simulink model "at3_2"  (R2020a)
settings: Solver=VariableStepAuto  StartTime=0.0  StopTime=3.5  RelTol=1e-3
model workspace (MAT data in the model file):
  T = [1  0  0  0; 0  1  0  0; 0  0  1  0; 0  0  0  1]
  bd = 5
  kd = 10
  md = 1
  myFd = [0; 0; 5; 0; 0; 0]
  mybot = SerialLink
  mybot.name = 'mybot'
  mybot.gravity = [0; 0; 9.81]
  mybot.base = SE3
  mybot.base.data = [1  0  0  0; 0  1  0  0; 0  0  1  0; 0  0  0  1]
  mybot.tool = SE3
  mybot.tool.data = [1  0  0  0; 0  1  0  0; 0  0  1  0; 0  0  0  1]
  mybot.fast = 0
  mybot.delay = 0.1
  mybot.loop = 0
  mybot.n = 6
  mybot.links(1) = Link
  mybot.links(1).theta = 0
  mybot.links(1).d = 0.29333
  mybot.links(1).alpha = -1.57079632679
  mybot.links(1).a = 0.26667
  mybot.links(1).jointtype = 'R'
  mybot.links(1).mdh = 0
  mybot.links(1).offset = 0
  mybot.links(1).flip = 0
  mybot.links(1).m = 60.981037037
  mybot.links(1).r = [-0.139481333333 0.0867106666667 -0.0425993333333]
  mybot.links(1).I = [0.756881647671  0.0380732803951  -0.104663306798; 0.0380732803951  1.31862233218  -0.0252104658436; -0.104663306798  -0.0252104658436  1.48229918249]
  mybot.links(1).Jm = 0
  mybot.links(1).B = 0
  mybot.links(1).Tc = [0 0]
  mybot.links(1).G = 0
  mybot.links(1).qlim = [-3.14159265359 3.14159265359]
  mybot.links(2) = Link
  mybot.links(2).theta = 0
  mybot.links(2).d = 0
  mybot.links(2).alpha = 0
  mybot.links(2).a = 0.666666666667
  mybot.links(2).jointtype = 'R'
  mybot.links(2).mdh = 0
  mybot.links(2).offset = -1.57079632679
  mybot.links(2).flip = 0
  mybot.links(2).m = 30.4687407407
  mybot.links(2).r = [-0.364482 0.031008 -0.203550666667]
  mybot.links(2).I = [0.445067283621  -0.108967727539  0.582977155556; -0.108967727539  5.764327397  -0.00631798241975; 0.582977155556  -0.00631798241975  5.74215637531]
  mybot.links(2).Jm = 0
  mybot.links(2).B = 0
  mybot.links(2).Tc = [0 0]
  mybot.links(2).G = 0
  mybot.links(2).qlim = [-1.24756134933 1.28316606607]
  mybot.links(3) = Link
  mybot.links(3).theta = 0
  mybot.links(3).d = 0
  mybot.links(3).alpha = -1.57079632679
  mybot.links(3).a = 0
  mybot.links(3).jointtype = 'R'
  mybot.links(3).mdh = 0
  mybot.links(3).offset = 0
  mybot.links(3).flip = 0
  mybot.links(3).m = 79.3111111111
  mybot.links(3).r = [-0.00110933333333 0.0488613333333 0.203686]
  mybot.links(3).I = [1.64625289455  -0.0104833337942  0.0982028045432; -0.0104833337942  1.62048570864  -0.0496952560988; 0.0982028045432  -0.0496952560988  0.173149863111]
  mybot.links(3).Jm = 0
  mybot.links(3).B = 0
  mybot.links(3).Tc = [0 0]
  mybot.links(3).G = 0
  mybot.links(3).qlim = [-3.56431139842 1.14807758196]
  mybot.links(4) = Link
  mybot.links(4).theta = 0
  mybot.links(4).d = 0.87133
  mybot.links(4).alpha = 1.57079632679
  mybot.links(4).a = 0
  mybot.links(4).jointtype = 'R'
  mybot.links(4).mdh = 0
  mybot.links(4).offset = 0
  mybot.links(4).flip = 0
  mybot.links(4).m = 7.42785185185
  mybot.links(4).r = [0 -0.114642 -0.0563753333333]
  mybot.links(4).I = [0.0760047099259  -0.00573300266667  8.43277695473e-05; -0.00573300266667  0.0244535510123  -0.000540736395062; 8.43277695473e-05  -0.000540736395062  0.0768069846914]
  mybot.links(4).Jm = 0
  mybot.links(4).B = 0
  mybot.links(4).Tc = [0 0]
  mybot.links(4).G = 0
  mybot.links(4).qlim = [-3.14159265359 3.14159265359]
  mybot.links(5) = Link
  mybot.links(5).theta = 0
  mybot.links(5).d = 0
  mybot.links(5).alpha = -1.57079632679
  mybot.links(5).a = 0
  mybot.links(5).jointtype = 'R'
  mybot.links(5).mdh = 0
  mybot.links(5).offset = 0
  mybot.links(5).flip = 0
  mybot.links(5).m = 3.22814814815
  mybot.links(5).r = [0 0.055874 0.009464]
  mybot.links(5).I = [0.0620193424856  -0.00336486123457  0.00258873902881; -0.00336486123457  0.0425072813827  -0.00932130199177; 0.00258873902881  -0.00932130199177  0.042955055144]
  mybot.links(5).Jm = 0
  mybot.links(5).B = 0
  mybot.links(5).Tc = [0 0]
  mybot.links(5).G = 0
  mybot.links(5).qlim = [-1.91986217719 1.91986217719]
  mybot.links(6) = Link
  mybot.links(6).theta = 0
  mybot.links(6).d = 0.40667
  mybot.links(6).alpha = 0
  mybot.links(6).a = 0
  mybot.links(6).jointtype = 'R'
  mybot.links(6).mdh = 0
  mybot.links(6).offset = 0
  mybot.links(6).flip = 0
  mybot.links(6).m = 0.993777777778
  mybot.links(6).r = [7.33333333333e-06 0.0546666666667 -0.0859013333333]
  mybot.links(6).I = [0.00060011417284  0  0; 0  0.000924736395062  0; 0  0  0.000554118716049]
  mybot.links(6).Jm = 0
  mybot.links(6).B = 0
  mybot.links(6).Tc = [0 0]
  mybot.links(6).G = 0
  mybot.links(6).qlim = [-3.14159265359 3.14159265359]
  mybot.mdh = 0
values from neighbouring files (symbols this model uses):
  Fd2 = [0 0 5 0 0 0]'    [main.m]
  Fd3 = [0 0 0 0 0 0]'    [main.m]
  m = [171.459 140.993 94.498 31.976 31.091 0.606]    [I.mat]    (also in main.m = [205.811,102.832,267.675,25.069,10.895,3.354]; maincircle.m = [205.811,102.832,267.675,25.069,10.895,3.354])
undefined symbols (not defined in the file or in its folder): X, Y, Z
libraries: sm_lib x76, nesl_utility x31, simulink_extras x21, roblocks x16, simulink x7
(part 1 of 3)
settings Model: PauseTimes=1.625  Creator=93548  LastModifiedBy=93548

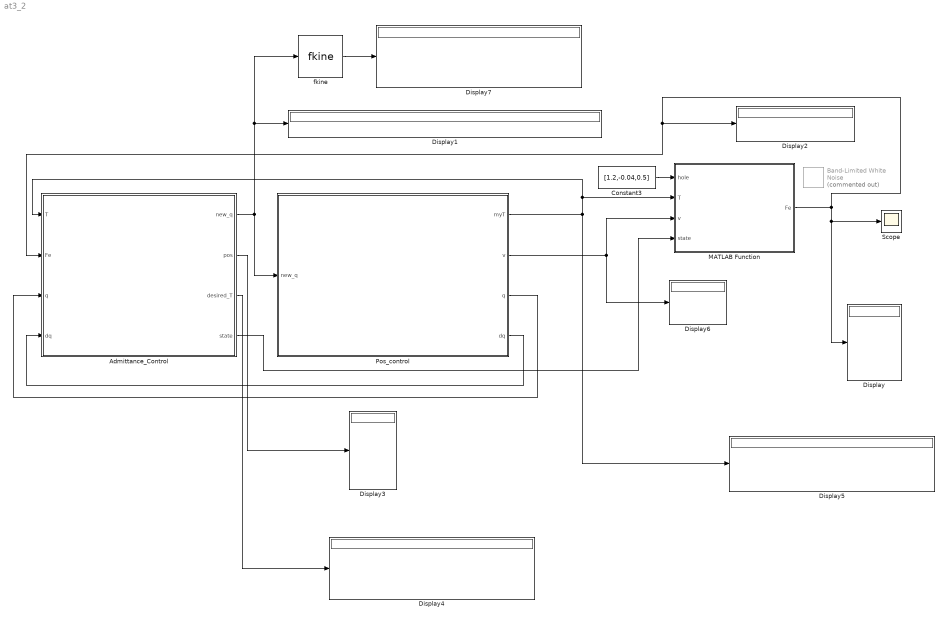
== system at3_2 ==
  Admittance_Control : Subsystem
  Band-Limited White Noise : simulink/Sources/Band-Limited White Noise  Commented=on  Cov=0.00001*ones(1,6)  Ts=0.01  seed=[23341 2221 2342 4533 53 123]
  Constant3 : Constant  Value=[1.2,-0.04,0.5]
  Display{,1..7} (8 alike) : Display
  MATLAB Function : MATLAB Function  TreatAsAtomicUnit=on
  Pos_control : Subsystem
  Scope : Scope
  fkine : roblocks/Arm/fkine  robot=mybot
  wires:
  Admittance_Control/3(desired_T) -> Display4/1
  Pos_control/3(q) -> Admittance_Control/3(q)
  MATLAB Function/1(Fe) -> Display2/1, Admittance_Control/2(Fe), Scope/1, Display/1
  Pos_control/1(myT) -> MATLAB Function/2(T), Admittance_Control/1(T), Display5/1
  Pos_control/4(dq) -> Admittance_Control/4(dq)
  Constant3/1 -> MATLAB Function/1(hole)
  Admittance_Control/1(new_q) -> Pos_control/1(new_q), fkine/1, Display1/1
  Admittance_Control/2(pos) -> Display3/1
  Pos_control/2(v) -> MATLAB Function/3(v), Display6/1
  fkine/1 -> Display7/1
  Admittance_Control/4(state) -> MATLAB Function/4(state)

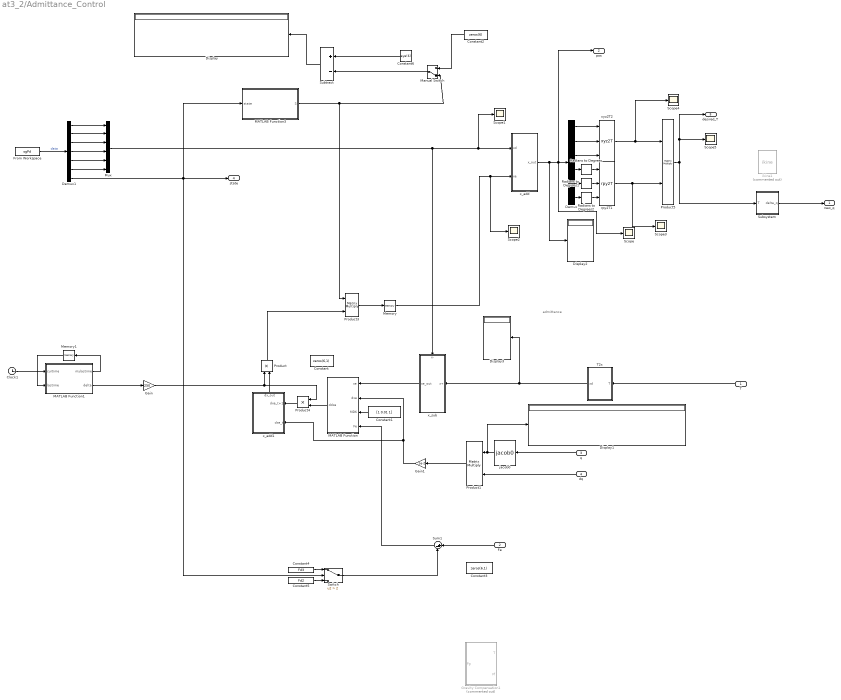
== system at3_2/Admittance_Control ==
  note: admittance
  T : Inport  InitFcn=T=eye(4)
  Fe : Inport  Port=2
  q : Inport  Port=3
  dq : Inport  Port=4
  Clock1 : Clock
  Constant : Constant  Value=zeros(6,1)
  Constant1 : Constant  Value=[1 0.01 1]
  Constant2 : Constant  Value=zeros(6)
  Constant3 : Constant  Value=zeros(6,1)
  Constant4 : Constant  Value=Fd3
  Constant5 : Constant  Value=Fd2
  Constant6 : Constant  Value=eye(6)
  Demux : Demux  Outputs=6
  Demux1 : Demux  Outputs=7
  Display{,1..3} (4 alike) : Display
  From Workspace : FromWorkspace  VariableName=sgPd
  Gain : Gain  Gain=250
  Gain1 : Gain  Gain=1e-2
  Gravity Compensation1 : MATLAB Function  Commented=on  TreatAsAtomicUnit=on
  MATLAB Function : MATLAB Function  TreatAsAtomicUnit=on
  MATLAB Function1 : MATLAB Function  TreatAsAtomicUnit=on
  MATLAB Function3 : MATLAB Function  TreatAsAtomicUnit=on
  Manual Switch : ManualSwitch  CurrentSetting=0
  Memory : Memory  InitialCondition=zeros(6,1)
  Memory1 : Memory
  Mux : Mux  Inputs=6
  Product : Product
  Product1 : Product  Multiplication=Matrix(*)
  Product3 : Product  Multiplication=Matrix(*)
  Product4 : Product
  Product5 : Product  Multiplication=Matrix(*)
  Radians to Degrees : simulink_extras/Transformations/Radians to Degrees
  Radians to Degrees1 : simulink_extras/Transformations/Radians to Degrees
  Radians to Degrees2 : simulink_extras/Transformations/Radians to Degrees
  Scope{,1..5} (6 alike) : Scope
  Subsystem : Subsystem
  Subtract : Sum  Inputs=+-
  Sum1 : Sum  Inputs=|+-
  Switch : Switch  Criteria=u2 > Threshold  Threshold=2
  T2x : Subsystem
  ikine1 : roblocks/Arm/ikine  Commented=on  robot=mybot  q0=zeros(6,1)  M=[1 1 1 1 1 1]  pinv=off  options={}
  "jacob0 " : roblocks/Arm/jacob0   robot=mybot
  rpy2T1 : roblocks/Toolbox/rpy2T  sequence=XYZ  degrees=off
  x_add : Subsystem
  x_add1 : Subsystem
      settings: PortSchema="{\"entries\":[{\"content\":{\"sides\":[{\"content\":{\"connectorIds\":[\"In1\",\"In2\"]},\"type\":\"ConnectorPlacement.EquallySpacedRectSide\",\"uuid\":\"360d4010-1b97-427a-9903-25c88b23e70b\"},{\"content\":{\"connectorIds\":[],\"side\":\"RIGHT\"},\"type\":\"ConnectorPlacement.EquallySpacedRectSide\",\"uuid\":\"9a31a209-5194-4c7d-8d7e-c14204494445\"},{\"content\":{\"connectorIds\":[\"Out1\"],\"side\":\"TOP\"},\"type\":\"ConnectorPlacement.EquallySpacedRectSide\",\"uuid\":\"bbbce9f7-61ee-4f1f-a5ce-85863fd91b3c\"}]},\"type\":\"ConnectorPlacement.EquallySpacedConnector\",\"uuid\":\"e93273eb-05a0-482b-8f1c-7b726ecfc3e6\"}],\"packageUris\":[\"http://schema.mathworks.com/mf0/Connector/19700101\"],\"version\":\"1.0\"}"
  x_sub : Subsystem
      settings: PortSchema="{\"entries\":[{\"content\":{\"sides\":[{\"content\":{\"connectorIds\":[\"In1\"]},\"type\":\"ConnectorPlacement.EquallySpacedRectSide\",\"uuid\":\"dec81ac2-0bd0-410d-a885-3af3e0ce6e73\"},{\"content\":{\"connectorIds\":[\"Out1\"],\"side\":\"RIGHT\"},\"type\":\"ConnectorPlacement.EquallySpacedRectSide\",\"uuid\":\"6534a841-e66b-4c1b-a3eb-8f152edb689c\"},{\"content\":{\"connectorIds\":[\"In2\"],\"side\":\"TOP\"},\"type\":\"ConnectorPlacement.EquallySpacedRectSide\",\"uuid\":\"16d8580e-7ffb-477c-bb08-41121949b294\"}]},\"type\":\"ConnectorPlacement.EquallySpacedConnector\",\"uuid\":\"cf84df31-fda1-43e7-8245-e4491d5279cc\"}],\"packageUris\":[\"http://schema.mathworks.com/mf0/Connector/19700101\"],\"version\":\"1.0\"}"
  xyz2T2 : roblocks/Toolbox/xyz2T
  new_q : Outport
  pos : Outport  Port=2
  desired_T : Outport  Port=3
  state : Outport  Port=4
  wires:
  Fe/1 -> Sum1/1
  rpy2T1/1 -> Product5/2, Scope3/1
  Demux/1 -> xyz2T2/1
  Demux/2 -> xyz2T2/2
  Demux/3 -> xyz2T2/3
  Demux/4 -> Radians to Degrees/1
  Demux/5 -> Radians to Degrees1/1
  Demux/6 -> Radians to Degrees2/1
  Constant6/1 -> Subtract/1
  T2x/1(xd) -> Display3/1, x_sub/1(x+)
  "jacob0 "/1 -> Display1/1, Product1/1
  x_sub/1(xe_out) -> MATLAB Function/1(xe)
  Constant1/1 -> MATLAB Function/3(MDK)
  MATLAB Function/1(ddxe) -> Product4/2
  x_add1/1(dx_out) -> Product/2
  Subtract/1 -> Display/1
  Mux/1 -> x_sub/2(x-), Scope1/1, x_add/1(xd)
  Manual Switch/1 -> Subtract/2
  MATLAB Function3/1(S) -> Manual Switch/2, Product3/1
  Constant2/1 -> Manual Switch/1
  T/1 -> T2x/1(T)
  Radians to Degrees/1 -> rpy2T1/1
  Radians to Degrees1/1 -> rpy2T1/2
  Radians to Degrees2/1 -> rpy2T1/3
  From Workspace/1 -> Demux1/1  "data"
  Demux1/6 -> Mux/6
  Demux1/5 -> Mux/5
  Demux1/3 -> Mux/3
  Demux1/4 -> Mux/4
  Demux1/2 -> Mux/2
  Demux1/1 -> Mux/1
  Demux1/7 -> MATLAB Function3/1(state), state/1, Switch/2
  x_add/1(x_out) -> Scope/1, Demux/1, pos/1, Display2/1
  Product5/1 -> Scope5/1, desired_T/1, Subsystem/1(T)
  Product/1 -> Product3/2
  q/1 -> "jacob0 "/1
  dq/1 -> Product1/2
  Product3/1 -> Memory/1
  Memory/1 -> Scope2/1, x_add/2(xe)
  Sum1/1 -> MATLAB Function/4(Fe)
  Constant4/1 -> Switch/1
  Constant5/1 -> Switch/3
  Switch/1 -> Sum1/2
  MATLAB Function1/2(delta) -> Gain/1
  MATLAB Function1/1(mylastime) -> Memory1/1
  Clock1/1 -> MATLAB Function1/1(curtime)
  Memory1/1 -> MATLAB Function1/2(lastime)
  Product4/1 -> x_add1/1(dxe_t+1)
  Subsystem/1(delta_q) -> new_q/1
  xyz2T2/1 -> Scope4/1, Product5/1
  Gain/1 -> Product4/1, Product/1
  Gain1/1 -> MATLAB Function/2(dxe), x_add1/2(dxe_t)
  Product1/1 -> Gain1/1

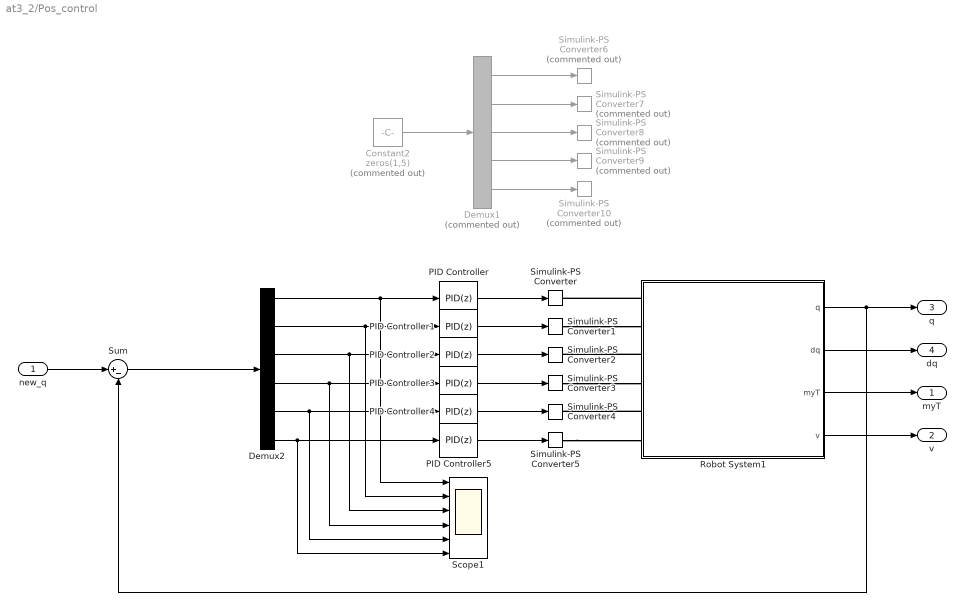
== system at3_2/Pos_control ==
  new_q : Inport
  Constant2 : Constant  Commented=on  Value=zeros(1,5)
  Demux1 : Demux  Commented=on  Outputs=5
  Demux2 : Demux  Outputs=6
  PID Controller : simulink/Continuous/PID Controller  Controller=PID  Form=Parallel  TimeDomain=Discrete-time  UseExternalTs=off  SampleTime=-1  IntegratorMethod=Forward Euler  FilterMethod=Forward Euler  ControllerParametersSource=internal  P=4465.98498018288  I=7608.36685462562  D=641.613681305102  UseFilter=on  N=345.506450530319  TunerSelectOption=Transfer Function Based (PID Tuner App)  InitialConditionSource=internal  InitialConditionForIntegrator=0  InitialConditionForFilter=0  DifferentiatorICPrevScaledInput=0  ExternalReset=none  TrackingMode=off  Kt=1  LimitOutput=off  UpperSaturationLimit=inf  LowerSaturationLimit=-inf  LinearizeAsGain=on  AntiWindupMode=none  Kb=1  POutMin=[]  POutMax=[]  IOutMin=[]  IOutMax=[]  DOutMin=[]  DOutMax=[]  NOutMin=[]  NOutMax=[]  SumOutMin=[]  SumOutMax=[]  SaturationOutMin=[]  SaturationOutMax=[]  PParamMin=[]  PParamMax=[]  IParamMin=[]  IParamMax=[]  DParamMin=[]  DParamMax=[]  NParamMin=[]  NParamMax=[]  KbParamMin=[]  KbParamMax=[]  KtParamMin=[]  KtParamMax=[]  KbOutMin=[]  KbOutMax=[]  KtOutMin=[]  KtOutMax=[]  IntegratorOutMin=[]  IntegratorOutMax=[]  FilterOutMin=[]  FilterOutMax=[]  SumI1OutMin=[]  SumI1OutMax=[]  SumI2OutMin=[]  SumI2OutMax=[]  SumI3OutMin=[]  SumI3OutMax=[]  SumI4OutMin=[]  SumI4OutMax=[]  SumDOutMin=[]  SumDOutMax=[]  DifferentiatorOutMin=[]  DifferentiatorOutMax=[]  FilterDiffOutCoefMin=[]  FilterDiffOutCoefMax=[]  ReciprocalOutMin=[]  ReciprocalOutMax=[]  SumDenOutMin=[]  SumDenOutMax=[]  SumNumOutMin=[]  SumNumOutMax=[]  DivideOutMin=[]  DivideOutMax=[]  UdiffTsProdOutMin=[]  UdiffTsProdOutMax=[]  NTsProdOutMin=[]  NTsProdOutMax=[]  UintegralTsProdOutMin=[]  UintegralTsProdOutMax=[]  UngainTsProdOutMin=[]  UngainTsProdOutMax=[]  IntegratorContinuousStateAttributes=''  IntegratorStateMustResolveToSignalObject=off  IntegratorRTWStateStorageClass=Auto  FilterContinuousStateAttributes=''  FilterStateMustResolveToSignalObject=off  FilterRTWStateStorageClass=Auto  ParallelPVariant=InternalParameters  IdealPVariant=Disabled  IVariant=InternalParameters  DVariant=InternalParameters  IntegratorVariant=Discrete  SatVariant=Disabled  AWVariant=Passthrough  PCopyVariant=Disabled  TRVariant=Disabled  FdbkBlocksVariant=Forward  IdealPFdbkVariant=Disabled  SatFdbkVariant=Disabled  DerivativeFilterVariant=ForwardEulerFilter  NVariant=InternalParameters  NCopyVariant=Disabled  FilterICVariant=InternalICsFilter  IntegratorICVariant=InternalICs  ExternalResetVariant=Disabled  TRSumVariant=Passthrough  SumFdbkVariant=Disabled  SumVariant=Sum_PID  TsampFilterVariant=InternalTs  TsampNgainVariant=Passthrough  TsampIntegralVariant=Passthrough
  PID Controller1 : simulink/Continuous/PID Controller  Controller=PID  Form=Parallel  TimeDomain=Discrete-time  UseExternalTs=off  SampleTime=-1  IntegratorMethod=Forward Euler  FilterMethod=Forward Euler  ControllerParametersSource=internal  P=16138.220391969  I=29003.8058546243  D=1312.1656601102  UseFilter=on  N=1517.01833251505  TunerSelectOption=Transfer Function Based (PID Tuner App)  InitialConditionSource=internal  InitialConditionForIntegrator=0  InitialConditionForFilter=0  DifferentiatorICPrevScaledInput=0  ExternalReset=none  TrackingMode=off  Kt=1  LimitOutput=off  UpperSaturationLimit=inf  LowerSaturationLimit=-inf  LinearizeAsGain=on  AntiWindupMode=none  Kb=1  POutMin=[]  POutMax=[]  IOutMin=[]  IOutMax=[]  DOutMin=[]  DOutMax=[]  NOutMin=[]  NOutMax=[]  SumOutMin=[]  SumOutMax=[]  SaturationOutMin=[]  SaturationOutMax=[]  PParamMin=[]  PParamMax=[]  IParamMin=[]  IParamMax=[]  DParamMin=[]  DParamMax=[]  NParamMin=[]  NParamMax=[]  KbParamMin=[]  KbParamMax=[]  KtParamMin=[]  KtParamMax=[]  KbOutMin=[]  KbOutMax=[]  KtOutMin=[]  KtOutMax=[]  IntegratorOutMin=[]  IntegratorOutMax=[]  FilterOutMin=[]  FilterOutMax=[]  SumI1OutMin=[]  SumI1OutMax=[]  SumI2OutMin=[]  SumI2OutMax=[]  SumI3OutMin=[]  SumI3OutMax=[]  SumI4OutMin=[]  SumI4OutMax=[]  SumDOutMin=[]  SumDOutMax=[]  DifferentiatorOutMin=[]  DifferentiatorOutMax=[]  FilterDiffOutCoefMin=[]  FilterDiffOutCoefMax=[]  ReciprocalOutMin=[]  ReciprocalOutMax=[]  SumDenOutMin=[]  SumDenOutMax=[]  SumNumOutMin=[]  SumNumOutMax=[]  DivideOutMin=[]  DivideOutMax=[]  UdiffTsProdOutMin=[]  UdiffTsProdOutMax=[]  NTsProdOutMin=[]  NTsProdOutMax=[]  UintegralTsProdOutMin=[]  UintegralTsProdOutMax=[]  UngainTsProdOutMin=[]  UngainTsProdOutMax=[]  IntegratorContinuousStateAttributes=''  IntegratorStateMustResolveToSignalObject=off  IntegratorRTWStateStorageClass=Auto  FilterContinuousStateAttributes=''  FilterStateMustResolveToSignalObject=off  FilterRTWStateStorageClass=Auto  ParallelPVariant=InternalParameters  IdealPVariant=Disabled  IVariant=InternalParameters  DVariant=InternalParameters  IntegratorVariant=Discrete  SatVariant=Disabled  AWVariant=Passthrough  PCopyVariant=Disabled  TRVariant=Disabled  FdbkBlocksVariant=Forward  IdealPFdbkVariant=Disabled  SatFdbkVariant=Disabled  DerivativeFilterVariant=ForwardEulerFilter  NVariant=InternalParameters  NCopyVariant=Disabled  FilterICVariant=InternalICsFilter  IntegratorICVariant=InternalICs  ExternalResetVariant=Disabled  TRSumVariant=Passthrough  SumFdbkVariant=Disabled  SumVariant=Sum_PID  TsampFilterVariant=InternalTs  TsampNgainVariant=Passthrough  TsampIntegralVariant=Passthrough
  PID Controller2 : simulink/Continuous/PID Controller  Controller=PID  Form=Parallel  TimeDomain=Discrete-time  UseExternalTs=off  SampleTime=-1  IntegratorMethod=Forward Euler  FilterMethod=Forward Euler  ControllerParametersSource=internal  P=1649.40066842326  I=2863.75247346737  D=182.018728238073  UseFilter=on  N=172.788597852014  TunerSelectOption=Transfer Function Based (PID Tuner App)  InitialConditionSource=internal  InitialConditionForIntegrator=0  InitialConditionForFilter=0  DifferentiatorICPrevScaledInput=0  ExternalReset=none  TrackingMode=off  Kt=1  LimitOutput=off  UpperSaturationLimit=inf  LowerSaturationLimit=-inf  LinearizeAsGain=on  AntiWindupMode=none  Kb=1  POutMin=[]  POutMax=[]  IOutMin=[]  IOutMax=[]  DOutMin=[]  DOutMax=[]  NOutMin=[]  NOutMax=[]  SumOutMin=[]  SumOutMax=[]  SaturationOutMin=[]  SaturationOutMax=[]  PParamMin=[]  PParamMax=[]  IParamMin=[]  IParamMax=[]  DParamMin=[]  DParamMax=[]  NParamMin=[]  NParamMax=[]  KbParamMin=[]  KbParamMax=[]  KtParamMin=[]  KtParamMax=[]  KbOutMin=[]  KbOutMax=[]  KtOutMin=[]  KtOutMax=[]  IntegratorOutMin=[]  IntegratorOutMax=[]  FilterOutMin=[]  FilterOutMax=[]  SumI1OutMin=[]  SumI1OutMax=[]  SumI2OutMin=[]  SumI2OutMax=[]  SumI3OutMin=[]  SumI3OutMax=[]  SumI4OutMin=[]  SumI4OutMax=[]  SumDOutMin=[]  SumDOutMax=[]  DifferentiatorOutMin=[]  DifferentiatorOutMax=[]  FilterDiffOutCoefMin=[]  FilterDiffOutCoefMax=[]  ReciprocalOutMin=[]  ReciprocalOutMax=[]  SumDenOutMin=[]  SumDenOutMax=[]  SumNumOutMin=[]  SumNumOutMax=[]  DivideOutMin=[]  DivideOutMax=[]  UdiffTsProdOutMin=[]  UdiffTsProdOutMax=[]  NTsProdOutMin=[]  NTsProdOutMax=[]  UintegralTsProdOutMin=[]  UintegralTsProdOutMax=[]  UngainTsProdOutMin=[]  UngainTsProdOutMax=[]  IntegratorContinuousStateAttributes=''  IntegratorStateMustResolveToSignalObject=off  IntegratorRTWStateStorageClass=Auto  FilterContinuousStateAttributes=''  FilterStateMustResolveToSignalObject=off  FilterRTWStateStorageClass=Auto  ParallelPVariant=InternalParameters  IdealPVariant=Disabled  IVariant=InternalParameters  DVariant=InternalParameters  IntegratorVariant=Discrete  SatVariant=Disabled  AWVariant=Passthrough  PCopyVariant=Disabled  TRVariant=Disabled  FdbkBlocksVariant=Forward  IdealPFdbkVariant=Disabled  SatFdbkVariant=Disabled  DerivativeFilterVariant=ForwardEulerFilter  NVariant=InternalParameters  NCopyVariant=Disabled  FilterICVariant=InternalICsFilter  IntegratorICVariant=InternalICs  ExternalResetVariant=Disabled  TRSumVariant=Passthrough  SumFdbkVariant=Disabled  SumVariant=Sum_PID  TsampFilterVariant=InternalTs  TsampNgainVariant=Passthrough  TsampIntegralVariant=Passthrough
  PID Controller3 : simulink/Continuous/PID Controller  Controller=PID  Form=Parallel  TimeDomain=Discrete-time  UseExternalTs=off  SampleTime=-1  IntegratorMethod=Forward Euler  FilterMethod=Forward Euler  ControllerParametersSource=internal  P=14.6989445468851  I=23.6851292927488  D=1.1771070717056  UseFilter=on  N=1533.69648335729  TunerSelectOption=Transfer Function Based (PID Tuner App)  InitialConditionSource=internal  InitialConditionForIntegrator=0  InitialConditionForFilter=0  DifferentiatorICPrevScaledInput=0  ExternalReset=none  TrackingMode=off  Kt=1  LimitOutput=off  UpperSaturationLimit=inf  LowerSaturationLimit=-inf  LinearizeAsGain=on  AntiWindupMode=none  Kb=1  POutMin=[]  POutMax=[]  IOutMin=[]  IOutMax=[]  DOutMin=[]  DOutMax=[]  NOutMin=[]  NOutMax=[]  SumOutMin=[]  SumOutMax=[]  SaturationOutMin=[]  SaturationOutMax=[]  PParamMin=[]  PParamMax=[]  IParamMin=[]  IParamMax=[]  DParamMin=[]  DParamMax=[]  NParamMin=[]  NParamMax=[]  KbParamMin=[]  KbParamMax=[]  KtParamMin=[]  KtParamMax=[]  KbOutMin=[]  KbOutMax=[]  KtOutMin=[]  KtOutMax=[]  IntegratorOutMin=[]  IntegratorOutMax=[]  FilterOutMin=[]  FilterOutMax=[]  SumI1OutMin=[]  SumI1OutMax=[]  SumI2OutMin=[]  SumI2OutMax=[]  SumI3OutMin=[]  SumI3OutMax=[]  SumI4OutMin=[]  SumI4OutMax=[]  SumDOutMin=[]  SumDOutMax=[]  DifferentiatorOutMin=[]  DifferentiatorOutMax=[]  FilterDiffOutCoefMin=[]  FilterDiffOutCoefMax=[]  ReciprocalOutMin=[]  ReciprocalOutMax=[]  SumDenOutMin=[]  SumDenOutMax=[]  SumNumOutMin=[]  SumNumOutMax=[]  DivideOutMin=[]  DivideOutMax=[]  UdiffTsProdOutMin=[]  UdiffTsProdOutMax=[]  NTsProdOutMin=[]  NTsProdOutMax=[]  UintegralTsProdOutMin=[]  UintegralTsProdOutMax=[]  UngainTsProdOutMin=[]  UngainTsProdOutMax=[]  IntegratorContinuousStateAttributes=''  IntegratorStateMustResolveToSignalObject=off  IntegratorRTWStateStorageClass=Auto  FilterContinuousStateAttributes=''  FilterStateMustResolveToSignalObject=off  FilterRTWStateStorageClass=Auto  ParallelPVariant=InternalParameters  IdealPVariant=Disabled  IVariant=InternalParameters  DVariant=InternalParameters  IntegratorVariant=Discrete  SatVariant=Disabled  AWVariant=Passthrough  PCopyVariant=Disabled  TRVariant=Disabled  FdbkBlocksVariant=Forward  IdealPFdbkVariant=Disabled  SatFdbkVariant=Disabled  DerivativeFilterVariant=ForwardEulerFilter  NVariant=InternalParameters  NCopyVariant=Disabled  FilterICVariant=InternalICsFilter  IntegratorICVariant=InternalICs  ExternalResetVariant=Disabled  TRSumVariant=Passthrough  SumFdbkVariant=Disabled  SumVariant=Sum_PID  TsampFilterVariant=InternalTs  TsampNgainVariant=Passthrough  TsampIntegralVariant=Passthrough
  PID Controller4 : simulink/Continuous/PID Controller  Controller=PID  Form=Parallel  TimeDomain=Discrete-time  UseExternalTs=off  SampleTime=-1  IntegratorMethod=Forward Euler  FilterMethod=Forward Euler  ControllerParametersSource=internal  P=98.6724069978625  I=118.426367034708  D=4.05904729962159  UseFilter=on  N=1784.33996524078  TunerSelectOption=Transfer Function Based (PID Tuner App)  InitialConditionSource=internal  InitialConditionForIntegrator=0  InitialConditionForFilter=0  DifferentiatorICPrevScaledInput=0  ExternalReset=none  TrackingMode=off  Kt=1  LimitOutput=off  UpperSaturationLimit=inf  LowerSaturationLimit=-inf  LinearizeAsGain=on  AntiWindupMode=none  Kb=1  POutMin=[]  POutMax=[]  IOutMin=[]  IOutMax=[]  DOutMin=[]  DOutMax=[]  NOutMin=[]  NOutMax=[]  SumOutMin=[]  SumOutMax=[]  SaturationOutMin=[]  SaturationOutMax=[]  PParamMin=[]  PParamMax=[]  IParamMin=[]  IParamMax=[]  DParamMin=[]  DParamMax=[]  NParamMin=[]  NParamMax=[]  KbParamMin=[]  KbParamMax=[]  KtParamMin=[]  KtParamMax=[]  KbOutMin=[]  KbOutMax=[]  KtOutMin=[]  KtOutMax=[]  IntegratorOutMin=[]  IntegratorOutMax=[]  FilterOutMin=[]  FilterOutMax=[]  SumI1OutMin=[]  SumI1OutMax=[]  SumI2OutMin=[]  SumI2OutMax=[]  SumI3OutMin=[]  SumI3OutMax=[]  SumI4OutMin=[]  SumI4OutMax=[]  SumDOutMin=[]  SumDOutMax=[]  DifferentiatorOutMin=[]  DifferentiatorOutMax=[]  FilterDiffOutCoefMin=[]  FilterDiffOutCoefMax=[]  ReciprocalOutMin=[]  ReciprocalOutMax=[]  SumDenOutMin=[]  SumDenOutMax=[]  SumNumOutMin=[]  SumNumOutMax=[]  DivideOutMin=[]  DivideOutMax=[]  UdiffTsProdOutMin=[]  UdiffTsProdOutMax=[]  NTsProdOutMin=[]  NTsProdOutMax=[]  UintegralTsProdOutMin=[]  UintegralTsProdOutMax=[]  UngainTsProdOutMin=[]  UngainTsProdOutMax=[]  IntegratorContinuousStateAttributes=''  IntegratorStateMustResolveToSignalObject=off  IntegratorRTWStateStorageClass=Auto  FilterContinuousStateAttributes=''  FilterStateMustResolveToSignalObject=off  FilterRTWStateStorageClass=Auto  ParallelPVariant=InternalParameters  IdealPVariant=Disabled  IVariant=InternalParameters  DVariant=InternalParameters  IntegratorVariant=Discrete  SatVariant=Disabled  AWVariant=Passthrough  PCopyVariant=Disabled  TRVariant=Disabled  FdbkBlocksVariant=Forward  IdealPFdbkVariant=Disabled  SatFdbkVariant=Disabled  DerivativeFilterVariant=ForwardEulerFilter  NVariant=InternalParameters  NCopyVariant=Disabled  FilterICVariant=InternalICsFilter  IntegratorICVariant=InternalICs  ExternalResetVariant=Disabled  TRSumVariant=Passthrough  SumFdbkVariant=Disabled  SumVariant=Sum_PID  TsampFilterVariant=InternalTs  TsampNgainVariant=Passthrough  TsampIntegralVariant=Passthrough
  PID Controller5 : simulink/Continuous/PID Controller  Controller=PID  Form=Parallel  TimeDomain=Discrete-time  UseExternalTs=off  SampleTime=-1  IntegratorMethod=Forward Euler  FilterMethod=Forward Euler  ControllerParametersSource=internal  P=1.57423793511941  I=4.99903335998905  D=0.109727091124155  UseFilter=on  N=1702.33251187192  TunerSelectOption=Transfer Function Based (PID Tuner App)  InitialConditionSource=internal  InitialConditionForIntegrator=0  InitialConditionForFilter=0  DifferentiatorICPrevScaledInput=0  ExternalReset=none  TrackingMode=off  Kt=1  LimitOutput=off  UpperSaturationLimit=inf  LowerSaturationLimit=-inf  LinearizeAsGain=on  AntiWindupMode=none  Kb=1  POutMin=[]  POutMax=[]  IOutMin=[]  IOutMax=[]  DOutMin=[]  DOutMax=[]  NOutMin=[]  NOutMax=[]  SumOutMin=[]  SumOutMax=[]  SaturationOutMin=[]  SaturationOutMax=[]  PParamMin=[]  PParamMax=[]  IParamMin=[]  IParamMax=[]  DParamMin=[]  DParamMax=[]  NParamMin=[]  NParamMax=[]  KbParamMin=[]  KbParamMax=[]  KtParamMin=[]  KtParamMax=[]  KbOutMin=[]  KbOutMax=[]  KtOutMin=[]  KtOutMax=[]  IntegratorOutMin=[]  IntegratorOutMax=[]  FilterOutMin=[]  FilterOutMax=[]  SumI1OutMin=[]  SumI1OutMax=[]  SumI2OutMin=[]  SumI2OutMax=[]  SumI3OutMin=[]  SumI3OutMax=[]  SumI4OutMin=[]  SumI4OutMax=[]  SumDOutMin=[]  SumDOutMax=[]  DifferentiatorOutMin=[]  DifferentiatorOutMax=[]  FilterDiffOutCoefMin=[]  FilterDiffOutCoefMax=[]  ReciprocalOutMin=[]  ReciprocalOutMax=[]  SumDenOutMin=[]  SumDenOutMax=[]  SumNumOutMin=[]  SumNumOutMax=[]  DivideOutMin=[]  DivideOutMax=[]  UdiffTsProdOutMin=[]  UdiffTsProdOutMax=[]  NTsProdOutMin=[]  NTsProdOutMax=[]  UintegralTsProdOutMin=[]  UintegralTsProdOutMax=[]  UngainTsProdOutMin=[]  UngainTsProdOutMax=[]  IntegratorContinuousStateAttributes=''  IntegratorStateMustResolveToSignalObject=off  IntegratorRTWStateStorageClass=Auto  FilterContinuousStateAttributes=''  FilterStateMustResolveToSignalObject=off  FilterRTWStateStorageClass=Auto  ParallelPVariant=InternalParameters  IdealPVariant=Disabled  IVariant=InternalParameters  DVariant=InternalParameters  IntegratorVariant=Discrete  SatVariant=Disabled  AWVariant=Passthrough  PCopyVariant=Disabled  TRVariant=Disabled  FdbkBlocksVariant=Forward  IdealPFdbkVariant=Disabled  SatFdbkVariant=Disabled  DerivativeFilterVariant=ForwardEulerFilter  NVariant=InternalParameters  NCopyVariant=Disabled  FilterICVariant=InternalICsFilter  IntegratorICVariant=InternalICs  ExternalResetVariant=Disabled  TRSumVariant=Passthrough  SumFdbkVariant=Disabled  SumVariant=Sum_PID  TsampFilterVariant=InternalTs  TsampNgainVariant=Passthrough  TsampIntegralVariant=Passthrough
  Robot System1 : Subsystem
  Scope1 : Scope  NumInputPorts=6
  Simulink-PS Converter{,1..5} (6 alike) : nesl_utility/Simulink-PS Converter  PhysicalDomain=network_engine_domain  SubClassName=ps_input  LeftPortType=input  RightPortType=output  PseudoPeriodic=off  Frequencies=[]  NoiseDistribution=none  NoiseParameters=[]  Unit=N*m  AffineConversion=off  FilteringAndDerivatives=filter  SimscapeFilterOrder=2  InputFilterTimeConstant=0.001  UdotUserProvided=0
  Simulink-PS Converter{6..10} (5 alike) : nesl_utility/Simulink-PS Converter  Commented=on  PhysicalDomain=network_engine_domain  SubClassName=ps_input  LeftPortType=input  RightPortType=output  PseudoPeriodic=off  Frequencies=[]  NoiseDistribution=none  NoiseParameters=[]  Unit=deg  AffineConversion=off  FilteringAndDerivatives=filter  SimscapeFilterOrder=2  InputFilterTimeConstant=0.001  UdotUserProvided=0
  Sum : Sum  Inputs=|+-
  myT : Outport
  v : Outport  Port=2
  q : Outport  Port=3
  dq : Outport  Port=4
  wires:
  Demux1/3 -> Simulink-PS Converter8/1
  Demux1/1 -> Simulink-PS Converter6/1
  Demux1/5 -> Simulink-PS Converter10/1
  Constant2/1 -> Demux1/1
  Demux1/4 -> Simulink-PS Converter9/1
  Demux1/2 -> Simulink-PS Converter7/1
  Robot System1/1(q) -> q/1, Sum/2
  Robot System1/2(dq) -> dq/1
  Robot System1/3(myT) -> myT/1
  Robot System1/4(v) -> v/1
  PID Controller2/1 -> Simulink-PS Converter2/1
  Demux2/4 -> PID Controller3/1, Scope1/4
  PID Controller4/1 -> Simulink-PS Converter4/1
  Demux2/6 -> PID Controller5/1, Scope1/6
  Demux2/2 -> PID Controller1/1, Scope1/2
  PID Controller1/1 -> Simulink-PS Converter1/1
  Demux2/1 -> PID Controller/1, Scope1/1
  Demux2/3 -> PID Controller2/1, Scope1/3
  PID Controller5/1 -> Simulink-PS Converter5/1
  PID Controller/1 -> Simulink-PS Converter/1
  Demux2/5 -> PID Controller4/1, Scope1/5
  PID Controller3/1 -> Simulink-PS Converter3/1
  new_q/1 -> Sum/1
  Sum/1 -> Demux2/1
  connections:
  Simulink-PS Converter5/RConn1 -- Robot System1/LConn6
  Robot System1/LConn5 -- Simulink-PS Converter4/RConn1
  Simulink-PS Converter3/RConn1 -- Robot System1/LConn4
  Robot System1/LConn3 -- Simulink-PS Converter2/RConn1
  Simulink-PS Converter1/RConn1 -- Robot System1/LConn2
  Robot System1/LConn1 -- Simulink-PS Converter/RConn1

== system at3_2/Admittance_Control/Subsystem ==
  T : Inport
  Constant3 : Constant  Value=zeros(6,1)
  MATLAB Function1 : MATLAB Function  TreatAsAtomicUnit=on
  delta_q : Outport
  wires:
  Constant3/1 -> MATLAB Function1/2(start)
  T/1 -> MATLAB Function1/1(T)
  MATLAB Function1/1(mytheta) -> delta_q/1  "delta_q"

== system at3_2/Admittance_Control/T2x ==
  T : Inport
  Mux : Mux  Inputs=6
  T2rpy : roblocks/Toolbox/T2rpy  sequence=XYZ  degrees=off
  T2xyz : roblocks/Toolbox/T2xyz
  xd : Outport
  wires:
  T2rpy/3 -> Mux/6
  T2rpy/2 -> Mux/5
  T2xyz/3 -> Mux/3
  Mux/1 -> xd/1
  T2xyz/2 -> Mux/2
  T/1 -> T2rpy/1, T2xyz/1
  T2xyz/1 -> Mux/1
  T2rpy/1 -> Mux/4

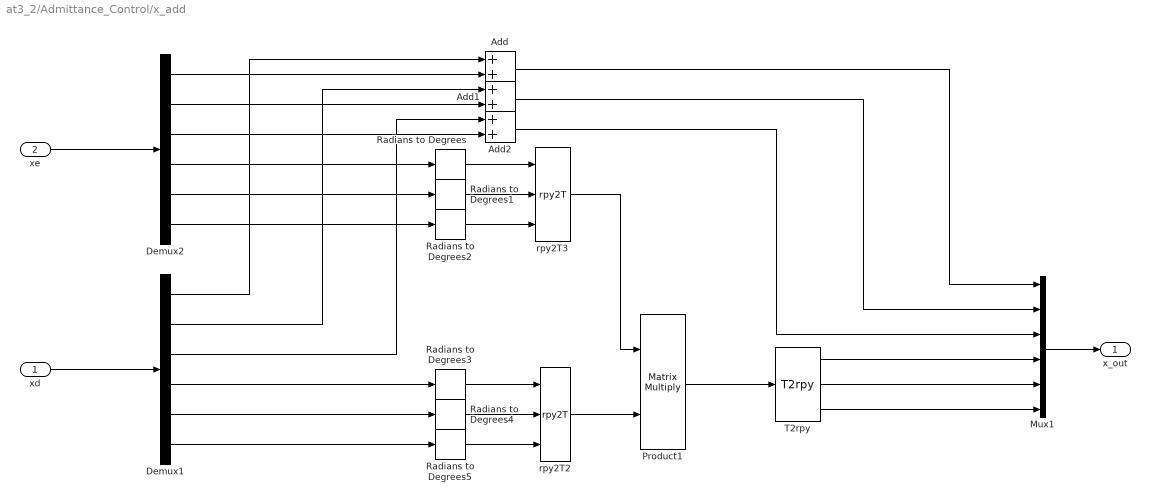
== system at3_2/Admittance_Control/x_add ==
  xd : Inport
  xe : Inport  Port=2
  Add : Sum
  Add1 : Sum
  Add2 : Sum
  Demux1 : Demux  Outputs=6
  Demux2 : Demux  Outputs=6
  Mux1 : Mux  Inputs=6
  Product1 : Product  Multiplication=Matrix(*)
  Radians to Degrees{,1..5} (6 alike) : simulink_extras/Transformations/Radians to Degrees
  T2rpy : roblocks/Toolbox/T2rpy  sequence=XYZ  degrees=off
  rpy2T2 : roblocks/Toolbox/rpy2T  sequence=XYZ  degrees=off
  rpy2T3 : roblocks/Toolbox/rpy2T  sequence=XYZ  degrees=off
  x_out : Outport
  wires:
  Demux2/6 -> Radians to Degrees2/1
  Mux1/1 -> x_out/1
  T2rpy/2 -> Mux1/5
  Demux1/1 -> Add/1
  xd/1 -> Demux1/1
  xe/1 -> Demux2/1
  Demux1/6 -> Radians to Degrees5/1
  Product1/1 -> T2rpy/1
  Add1/1 -> Mux1/2
  Demux1/3 -> Add2/1
  Demux1/2 -> Add1/1
  Add/1 -> Mux1/1
  Demux2/4 -> Radians to Degrees/1
  Demux2/2 -> Add1/2
  Demux2/3 -> Add2/2
  Add2/1 -> Mux1/3
  Demux2/5 -> Radians to Degrees1/1
  Demux2/1 -> Add/2
  Demux1/5 -> Radians to Degrees4/1
  Demux1/4 -> Radians to Degrees3/1
  T2rpy/1 -> Mux1/4
  T2rpy/3 -> Mux1/6
  rpy2T2/1 -> Product1/2
  rpy2T3/1 -> Product1/1
  Radians to Degrees/1 -> rpy2T3/1
  Radians to Degrees1/1 -> rpy2T3/2
  Radians to Degrees2/1 -> rpy2T3/3
  Radians to Degrees3/1 -> rpy2T2/1
  Radians to Degrees4/1 -> rpy2T2/2
  Radians to Degrees5/1 -> rpy2T2/3

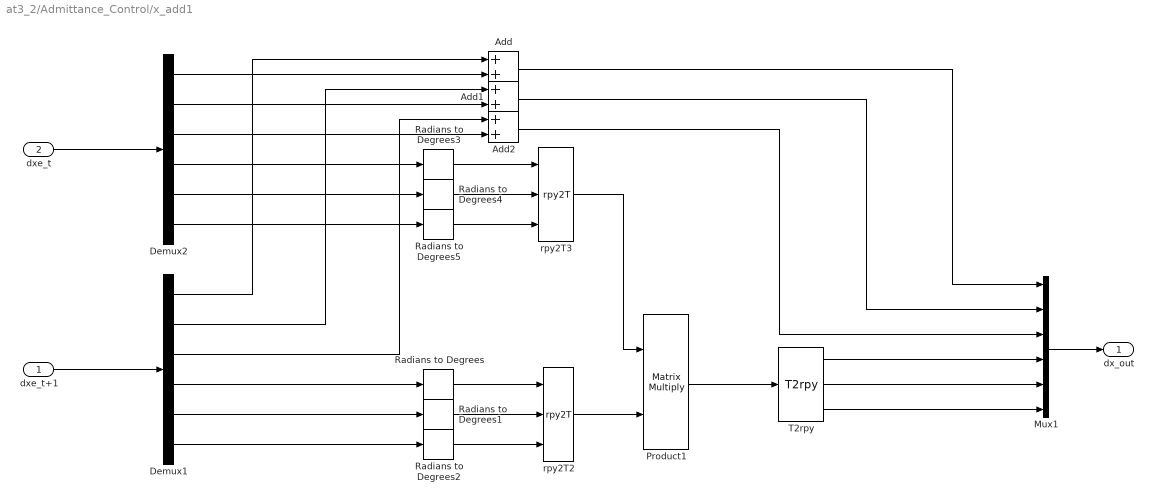
== system at3_2/Admittance_Control/x_add1 ==
  dxe_t+1 : Inport
  dxe_t : Inport  Port=2
  Add : Sum
  Add1 : Sum
  Add2 : Sum
  Demux1 : Demux  Outputs=6
  Demux2 : Demux  Outputs=6
  Mux1 : Mux  Inputs=6
  Product1 : Product  Multiplication=Matrix(*)
  Radians to Degrees{,1..5} (6 alike) : simulink_extras/Transformations/Radians to Degrees
  T2rpy : roblocks/Toolbox/T2rpy  sequence=XYZ  degrees=off
  rpy2T2 : roblocks/Toolbox/rpy2T  sequence=XYZ  degrees=off
  rpy2T3 : roblocks/Toolbox/rpy2T  sequence=XYZ  degrees=off
  dx_out : Outport
  wires:
  rpy2T3/1 -> Product1/1
  rpy2T2/1 -> Product1/2
  T2rpy/3 -> Mux1/6
  T2rpy/1 -> Mux1/4
  Demux1/4 -> Radians to Degrees/1
  Demux1/5 -> Radians to Degrees1/1
  Demux2/1 -> Add/2
  Demux2/5 -> Radians to Degrees4/1
  Add2/1 -> Mux1/3
  Demux2/3 -> Add2/2
  Demux2/2 -> Add1/2
  Demux2/4 -> Radians to Degrees3/1
  Add/1 -> Mux1/1
  Demux1/2 -> Add1/1
  Demux1/3 -> Add2/1
  Add1/1 -> Mux1/2
  Product1/1 -> T2rpy/1
  Demux1/6 -> Radians to Degrees2/1
  dxe_t/1 -> Demux2/1
  dxe_t+1/1 -> Demux1/1
  Demux1/1 -> Add/1
  T2rpy/2 -> Mux1/5
  Mux1/1 -> dx_out/1
  Demux2/6 -> Radians to Degrees5/1
  Radians to Degrees/1 -> rpy2T2/1
  Radians to Degrees1/1 -> rpy2T2/2
  Radians to Degrees2/1 -> rpy2T2/3
  Radians to Degrees3/1 -> rpy2T3/1
  Radians to Degrees4/1 -> rpy2T3/2
  Radians to Degrees5/1 -> rpy2T3/3

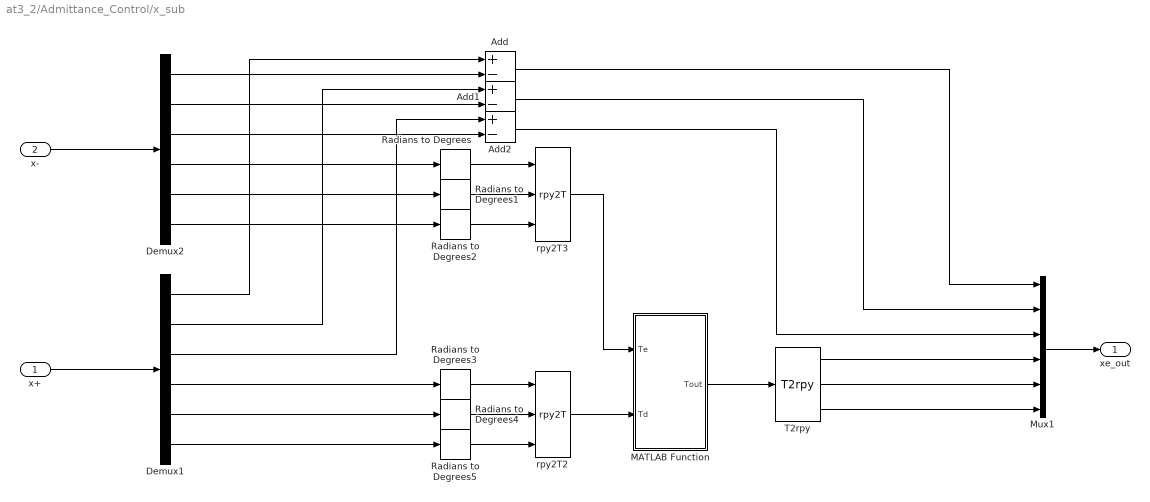
== system at3_2/Admittance_Control/x_sub ==
  x+ : Inport
  x- : Inport  Port=2
  Add : Sum  Inputs=+-
  Add1 : Sum  Inputs=+-
  Add2 : Sum  Inputs=+-
  Demux1 : Demux  Outputs=6
  Demux2 : Demux  Outputs=6
  MATLAB Function : MATLAB Function  TreatAsAtomicUnit=on
  Mux1 : Mux  Inputs=6
  Radians to Degrees{,1..5} (6 alike) : simulink_extras/Transformations/Radians to Degrees
  T2rpy : roblocks/Toolbox/T2rpy  sequence=XYZ  degrees=off
  rpy2T2 : roblocks/Toolbox/rpy2T  sequence=XYZ  degrees=off
  rpy2T3 : roblocks/Toolbox/rpy2T  sequence=XYZ  degrees=off
  xe_out : Outport
  wires:
  T2rpy/3 -> Mux1/6
  T2rpy/1 -> Mux1/4
  Demux1/4 -> Radians to Degrees3/1
  Demux1/5 -> Radians to Degrees4/1
  Demux2/1 -> Add/2
  Demux2/5 -> Radians to Degrees1/1
  Add2/1 -> Mux1/3
  Demux2/3 -> Add2/2
  Demux2/2 -> Add1/2
  Demux2/4 -> Radians to Degrees/1
  Add/1 -> Mux1/1
  Demux1/2 -> Add1/1
  Demux1/3 -> Add2/1
  Add1/1 -> Mux1/2
  Demux1/6 -> Radians to Degrees5/1
  x-/1 -> Demux2/1
  x+/1 -> Demux1/1
  Demux1/1 -> Add/1
  T2rpy/2 -> Mux1/5
  Mux1/1 -> xe_out/1
  Demux2/6 -> Radians to Degrees2/1
  rpy2T2/1 -> MATLAB Function/2(Td)
  MATLAB Function/1(Tout) -> T2rpy/1
  rpy2T3/1 -> MATLAB Function/1(Te)
  Radians to Degrees/1 -> rpy2T3/1
  Radians to Degrees1/1 -> rpy2T3/2
  Radians to Degrees2/1 -> rpy2T3/3
  Radians to Degrees3/1 -> rpy2T2/1
  Radians to Degrees4/1 -> rpy2T2/2
  Radians to Degrees5/1 -> rpy2T2/3

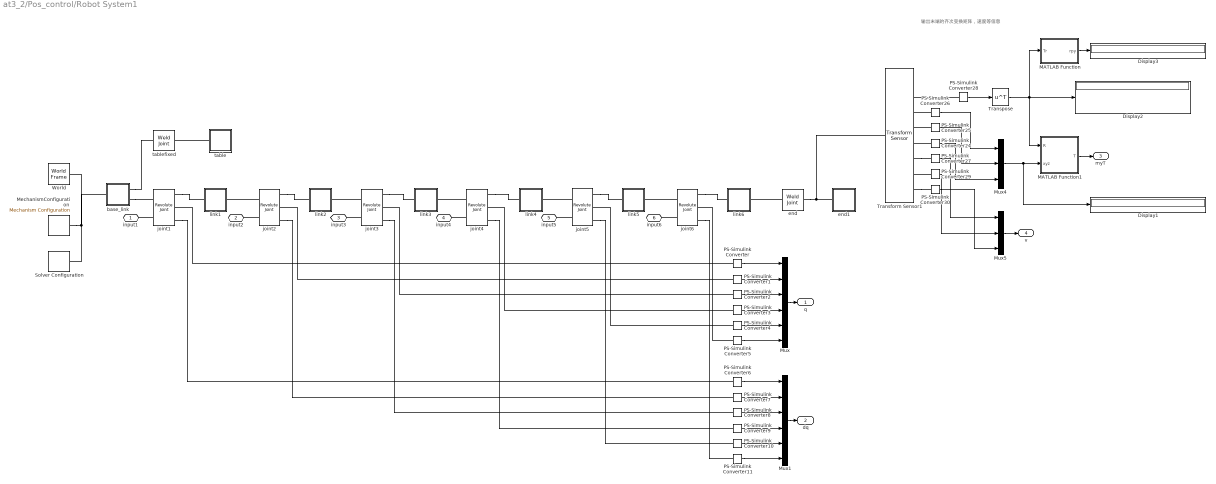
== system at3_2/Pos_control/Robot System1 ==
  note: 输出末端的齐次变换矩阵，速度等信息
  Display1 : Display
  Display2 : Display
  Display3 : Display
  MATLAB Function : MATLAB Function  TreatAsAtomicUnit=on
  MATLAB Function1 : MATLAB Function  TreatAsAtomicUnit=on
  MechanismConfiguration : sm_lib/Utilities/Mechanism Configuration  UniformGravity=Constant  GravityVector=[0, 0, -9.81]  GravityUnits=m/s^2  LinearizationDelta=0.001
  Mux : Mux  Inputs=6
  Mux1 : Mux  Inputs=6
  Mux4 : Mux  Inputs=3
  Mux5 : Mux  Inputs=3
  PS-Simulink Converter{,1..5} (6 alike) : nesl_utility/PS-Simulink Converter  PhysicalDomain=network_engine_domain  SubClassName=ps_output  LeftPortType=input  RightPortType=output  PseudoPeriodic=off  Frequencies=[]  Unit=rad  AffineConversion=off
  PS-Simulink Converter{6..11} (6 alike) : nesl_utility/PS-Simulink Converter  PhysicalDomain=network_engine_domain  SubClassName=ps_output  LeftPortType=input  RightPortType=output  PseudoPeriodic=off  Frequencies=[]  Unit=rad/s  AffineConversion=off
  PS-Simulink Converter24 : nesl_utility/PS-Simulink Converter  PhysicalDomain=network_engine_domain  SubClassName=ps_output  LeftPortType=input  RightPortType=output  PseudoPeriodic=off  Frequencies=[]  Unit=m  AffineConversion=off
  PS-Simulink Converter25 : nesl_utility/PS-Simulink Converter  PhysicalDomain=network_engine_domain  SubClassName=ps_output  LeftPortType=input  RightPortType=output  PseudoPeriodic=off  Frequencies=[]  Unit=m  AffineConversion=off
  PS-Simulink Converter26 : nesl_utility/PS-Simulink Converter  PhysicalDomain=network_engine_domain  SubClassName=ps_output  LeftPortType=input  RightPortType=output  PseudoPeriodic=off  Frequencies=[]  Unit=m  AffineConversion=off
  PS-Simulink Converter27 : nesl_utility/PS-Simulink Converter  PhysicalDomain=network_engine_domain  SubClassName=ps_output  LeftPortType=input  RightPortType=output  PseudoPeriodic=off  Frequencies=[]  Unit=m/s  AffineConversion=off
  PS-Simulink Converter28 : nesl_utility/PS-Simulink Converter  PhysicalDomain=network_engine_domain  SubClassName=ps_output  LeftPortType=input  RightPortType=output  PseudoPeriodic=off  Frequencies=[]  Unit=inherit  AffineConversion=off
  PS-Simulink Converter29 : nesl_utility/PS-Simulink Converter  PhysicalDomain=network_engine_domain  SubClassName=ps_output  LeftPortType=input  RightPortType=output  PseudoPeriodic=off  Frequencies=[]  Unit=m/s  AffineConversion=off
  PS-Simulink Converter30 : nesl_utility/PS-Simulink Converter  PhysicalDomain=network_engine_domain  SubClassName=ps_output  LeftPortType=input  RightPortType=output  PseudoPeriodic=off  Frequencies=[]  Unit=m/s  AffineConversion=off
  Solver Configuration : nesl_utility/Solver Configuration  PhysicalDomain=network_engine_domain  SubClassName=solver  LeftPortType=input  RightPortType=generic  Tones=[]  Harmonics=[]  SimulateNoise=off  Profile=off  UseLocalSampling=off  EnableSwitchedLinearOptims=on  FrequencyDomain=off  UseCCode=off  RelTol=0.001  AbsTol=1e-06  MinStep=1e-09  ToWorkspace=off  RevertToSquareIcSolve=off  NumHomotopyIterations=100  PhasorMode=off  PhasorModeNumHarmonics=1  DoDC=off  ResidualTolerance=1e-09  UseLocalSolver=off  LocalSolverChoice=NE_BACKWARD_EULER_ADVANCER  LocalSolverSampleTime=0.001  DoFixedCost=off  MaxNonlinIter=3  MaxModeIter=2  LinearAlgebra=auto  EquationFormulation=NE_TIME_EF  DelaysMemoryBudget=1024  AutomaticFiltering=on  FilteringTimeConstant=0.001  PartitionStorageMethod=AS_NEEDED  PartitionMemoryBudget=1024  PartitionMethod=ROBUST
  Transform Sensor1 : sm_lib/Frames and Transforms/Transform Sensor  MeasurementFrame=World  SenseAngle=off  SenseAxis=off  SenseAngle1=off  SenseAngle2=off  SenseAngle3=off  SenseQ=off  SenseR=on  SenseOmegaX=off  SenseOmegaY=off  SenseOmegaZ=off  SenseOmega1=off  SenseOmega2=off  SenseOmega3=off  SenseQDot=off  SenseRDot=off  SenseAlphaX=off  SenseAlphaY=off  SenseAlphaZ=off  SenseAlpha1=off  SenseAlpha2=off  SenseAlpha3=off  SenseQDDot=off  SenseRDDot=off  SenseX=on  SenseY=on  SenseZ=on  SenseRad=off  SenseAzim=off  SenseDist=off  SenseInc=off  SenseXDot=on  SenseYDot=on  SenseZDot=on  SenseRadDot=off  SenseAzimDot=off  SenseDistDot=off  SenseIncDot=off  SenseXDDot=off  SenseYDDot=off  SenseZDDot=off  SenseRadDDot=off  SenseAzimDDot=off  SenseDistDDot=off  SenseIncDDot=off
  Transpose : Math  Operator=transpose  SaturateOnIntegerOverflow=on
  World : sm_lib/Frames and Transforms/World Frame
  base_link : Subsystem
  end : sm_lib/Joints/Weld Joint  JointMode=Normal  SenseConstraintForce=off  SenseConstraintForceX=off  SenseConstraintForceY=off  SenseConstraintForceZ=off  SenseConstraintTorque=off  SenseConstraintTorqueX=off  SenseConstraintTorqueY=off  SenseConstraintTorqueZ=off  SenseTotalForce=off  SenseTotalForceX=off  SenseTotalForceY=off  SenseTotalForceZ=off  SenseTotalTorque=off  SenseTotalTorqueX=off  SenseTotalTorqueY=off  SenseTotalTorqueZ=off  CompositeWrenchDir=FollowerOnBase  CompositeWrenchFrame=BaseFrame
  end1 : Subsystem
  joint1 : sm_lib/Joints/Revolute Joint  JointMode=Normal  SenseConstraintForce=off  SenseConstraintForceX=off  SenseConstraintForceY=off  SenseConstraintForceZ=off  SenseConstraintTorque=off  SenseConstraintTorqueX=off  SenseConstraintTorqueY=off  SenseConstraintTorqueZ=off  SenseTotalForce=off  SenseTotalForceX=off  SenseTotalForceY=off  SenseTotalForceZ=off  SenseTotalTorque=off  SenseTotalTorqueX=off  SenseTotalTorqueY=off  SenseTotalTorqueZ=off  CompositeWrenchDir=FollowerOnBase  CompositeWrenchFrame=BaseFrame  EquilibriumPosition=0  EquilibriumPositionUnits=deg  SpringStiffness=0  SpringStiffnessUnits=N*m/deg  DampingCoefficient=0  DampingCoefficientUnits=m^2*kg/s/rad  TorqueActuationMode=InputTorque  MotionActuationMode=ComputedMotion  SensePosition=on  SenseVelocity=on  SenseAcceleration=off  SenseTorqueForce=off  SenseLowerLimitTorqueForce=off  SenseUpperLimitTorqueForce=off  LowerLimitSpecify=on  LowerLimitBound=-3.1416  LowerLimitBoundUnits=rad  LowerLimitStiffness=1e4  LowerLimitStiffnessUnits=N*m/deg  LowerLimitDamping=10  LowerLimitDampingUnits=N*m/(deg/s)  LowerLimitTransitionRegionWidth=0.1  LowerLimitTransitionRegionWidthUnits=deg  UpperLimitSpecify=on  UpperLimitBound=3.1416  UpperLimitBoundUnits=rad  UpperLimitStiffness=1e4  UpperLimitStiffnessUnits=N*m/deg  UpperLimitDamping=10  UpperLimitDampingUnits=N*m/(deg/s)  UpperLimitTransitionRegionWidth=0.1  UpperLimitTransitionRegionWidthUnits=deg  PositionTargetSpecify=on  PositionTargetPriority=High  PositionTargetValue=0  PositionTargetValueUnits=rad  VelocityTargetSpecify=off  VelocityTargetPriority=High  VelocityTargetValue=0  VelocityTargetValueUnits=deg/s
  joint2 : sm_lib/Joints/Revolute Joint  JointMode=Normal  SenseConstraintForce=off  SenseConstraintForceX=off  SenseConstraintForceY=off  SenseConstraintForceZ=off  SenseConstraintTorque=off  SenseConstraintTorqueX=off  SenseConstraintTorqueY=off  SenseConstraintTorqueZ=off  SenseTotalForce=off  SenseTotalForceX=off  SenseTotalForceY=off  SenseTotalForceZ=off  SenseTotalTorque=off  SenseTotalTorqueX=off  SenseTotalTorqueY=off  SenseTotalTorqueZ=off  CompositeWrenchDir=FollowerOnBase  CompositeWrenchFrame=BaseFrame  EquilibriumPosition=0  EquilibriumPositionUnits=deg  SpringStiffness=0  SpringStiffnessUnits=N*m/deg  DampingCoefficient=0  DampingCoefficientUnits=m^2*kg/s/rad  TorqueActuationMode=InputTorque  MotionActuationMode=ComputedMotion  SensePosition=on  SenseVelocity=on  SenseAcceleration=off  SenseTorqueForce=off  SenseLowerLimitTorqueForce=off  SenseUpperLimitTorqueForce=off  LowerLimitSpecify=on  LowerLimitBound=-1.2476  LowerLimitBoundUnits=rad  LowerLimitStiffness=1e4  LowerLimitStiffnessUnits=N*m/deg  LowerLimitDamping=10  LowerLimitDampingUnits=N*m/(deg/s)  LowerLimitTransitionRegionWidth=0.1  LowerLimitTransitionRegionWidthUnits=deg  UpperLimitSpecify=on  UpperLimitBound=1.2832  UpperLimitBoundUnits=rad  UpperLimitStiffness=1e4  UpperLimitStiffnessUnits=N*m/deg  UpperLimitDamping=10  UpperLimitDampingUnits=N*m/(deg/s)  UpperLimitTransitionRegionWidth=0.1  UpperLimitTransitionRegionWidthUnits=deg  PositionTargetSpecify=on  PositionTargetPriority=High  PositionTargetValue=0.0953  PositionTargetValueUnits=rad  VelocityTargetSpecify=off  VelocityTargetPriority=High  VelocityTargetValue=0  VelocityTargetValueUnits=deg/s
  joint3 : sm_lib/Joints/Revolute Joint  JointMode=Normal  SenseConstraintForce=off  SenseConstraintForceX=off  SenseConstraintForceY=off  SenseConstraintForceZ=off  SenseConstraintTorque=off  SenseConstraintTorqueX=off  SenseConstraintTorqueY=off  SenseConstraintTorqueZ=off  SenseTotalForce=off  SenseTotalForceX=off  SenseTotalForceY=off  SenseTotalForceZ=off  SenseTotalTorque=off  SenseTotalTorqueX=off  SenseTotalTorqueY=off  SenseTotalTorqueZ=off  CompositeWrenchDir=FollowerOnBase  CompositeWrenchFrame=BaseFrame  EquilibriumPosition=0  EquilibriumPositionUnits=deg  SpringStiffness=0  SpringStiffnessUnits=N*m/deg  DampingCoefficient=0  DampingCoefficientUnits=m^2*kg/s/rad  TorqueActuationMode=InputTorque  MotionActuationMode=ComputedMotion  SensePosition=on  SenseVelocity=on  SenseAcceleration=off  SenseTorqueForce=off  SenseLowerLimitTorqueForce=off  SenseUpperLimitTorqueForce=off  LowerLimitSpecify=on  LowerLimitBound=-3.5643  LowerLimitBoundUnits=rad  LowerLimitStiffness=1e4  LowerLimitStiffnessUnits=N*m/deg  LowerLimitDamping=10  LowerLimitDampingUnits=N*m/(deg/s)  LowerLimitTransitionRegionWidth=0.1  LowerLimitTransitionRegionWidthUnits=deg  UpperLimitSpecify=on  UpperLimitBound=1.1481  UpperLimitBoundUnits=rad  UpperLimitStiffness=1e4  UpperLimitStiffnessUnits=N*m/deg  UpperLimitDamping=10  UpperLimitDampingUnits=N*m/(deg/s)  UpperLimitTransitionRegionWidth=0.1  UpperLimitTransitionRegionWidthUnits=deg  PositionTargetSpecify=on  PositionTargetPriority=High  PositionTargetValue=-0.1523  PositionTargetValueUnits=rad  VelocityTargetSpecify=off  VelocityTargetPriority=High  VelocityTargetValue=0  VelocityTargetValueUnits=deg/s
  joint4 : sm_lib/Joints/Revolute Joint  JointMode=Normal  SenseConstraintForce=off  SenseConstraintForceX=off  SenseConstraintForceY=off  SenseConstraintForceZ=off  SenseConstraintTorque=off  SenseConstraintTorqueX=off  SenseConstraintTorqueY=off  SenseConstraintTorqueZ=off  SenseTotalForce=off  SenseTotalForceX=off  SenseTotalForceY=off  SenseTotalForceZ=off  SenseTotalTorque=off  SenseTotalTorqueX=off  SenseTotalTorqueY=off  SenseTotalTorqueZ=off  CompositeWrenchDir=FollowerOnBase  CompositeWrenchFrame=BaseFrame  EquilibriumPosition=0  EquilibriumPositionUnits=deg  SpringStiffness=0  SpringStiffnessUnits=N*m/deg  DampingCoefficient=0  DampingCoefficientUnits=m^2*kg/s/rad  TorqueActuationMode=InputTorque  MotionActuationMode=ComputedMotion  SensePosition=on  SenseVelocity=on  SenseAcceleration=off  SenseTorqueForce=off  SenseLowerLimitTorqueForce=off  SenseUpperLimitTorqueForce=off  LowerLimitSpecify=on  LowerLimitBound=-3.1416  LowerLimitBoundUnits=rad  LowerLimitStiffness=1e4  LowerLimitStiffnessUnits=N*m/deg  LowerLimitDamping=10  LowerLimitDampingUnits=N*m/(deg/s)  LowerLimitTransitionRegionWidth=0.1  LowerLimitTransitionRegionWidthUnits=deg  UpperLimitSpecify=on  UpperLimitBound=3.1416  UpperLimitBoundUnits=rad  UpperLimitStiffness=1e4  UpperLimitStiffnessUnits=N*m/deg  UpperLimitDamping=10  UpperLimitDampingUnits=N*m/(deg/s)  UpperLimitTransitionRegionWidth=0.1  UpperLimitTransitionRegionWidthUnits=deg  PositionTargetSpecify=on  PositionTargetPriority=High  PositionTargetValue=0  PositionTargetValueUnits=rad  VelocityTargetSpecify=off  VelocityTargetPriority=High  VelocityTargetValue=0  VelocityTargetValueUnits=deg/s
  joint5 : sm_lib/Joints/Revolute Joint  JointMode=Normal  SenseConstraintForce=off  SenseConstraintForceX=off  SenseConstraintForceY=off  SenseConstraintForceZ=off  SenseConstraintTorque=off  SenseConstraintTorqueX=off  SenseConstraintTorqueY=off  SenseConstraintTorqueZ=off  SenseTotalForce=off  SenseTotalForceX=off  SenseTotalForceY=off  SenseTotalForceZ=off  SenseTotalTorque=off  SenseTotalTorqueX=off  SenseTotalTorqueY=off  SenseTotalTorqueZ=off  CompositeWrenchDir=FollowerOnBase  CompositeWrenchFrame=BaseFrame  EquilibriumPosition=0  EquilibriumPositionUnits=deg  SpringStiffness=0  SpringStiffnessUnits=N*m/deg  DampingCoefficient=0  DampingCoefficientUnits=m^2*kg/s/rad  TorqueActuationMode=InputTorque  MotionActuationMode=ComputedMotion  SensePosition=on  SenseVelocity=on  SenseAcceleration=off  SenseTorqueForce=off  SenseLowerLimitTorqueForce=off  SenseUpperLimitTorqueForce=off  LowerLimitSpecify=on  LowerLimitBound=-1.92  LowerLimitBoundUnits=rad  LowerLimitStiffness=1e4  LowerLimitStiffnessUnits=N*m/deg  LowerLimitDamping=10  LowerLimitDampingUnits=N*m/(deg/s)  LowerLimitTransitionRegionWidth=0.1  LowerLimitTransitionRegionWidthUnits=deg  UpperLimitSpecify=on  UpperLimitBound=1.92  UpperLimitBoundUnits=rad  UpperLimitStiffness=1e4  UpperLimitStiffnessUnits=N*m/deg  UpperLimitDamping=10  UpperLimitDampingUnits=N*m/(deg/s)  UpperLimitTransitionRegionWidth=0.1  UpperLimitTransitionRegionWidthUnits=deg  PositionTargetSpecify=on  PositionTargetPriority=High  PositionTargetValue=1.6279  PositionTargetValueUnits=rad  VelocityTargetSpecify=off  VelocityTargetPriority=High  VelocityTargetValue=0  VelocityTargetValueUnits=deg/s
  joint6 : sm_lib/Joints/Revolute Joint  JointMode=Normal  SenseConstraintForce=off  SenseConstraintForceX=off  SenseConstraintForceY=off  SenseConstraintForceZ=off  SenseConstraintTorque=off  SenseConstraintTorqueX=off  SenseConstraintTorqueY=off  SenseConstraintTorqueZ=off  SenseTotalForce=off  SenseTotalForceX=off  SenseTotalForceY=off  SenseTotalForceZ=off  SenseTotalTorque=off  SenseTotalTorqueX=off  SenseTotalTorqueY=off  SenseTotalTorqueZ=off  CompositeWrenchDir=FollowerOnBase  CompositeWrenchFrame=BaseFrame  EquilibriumPosition=0  EquilibriumPositionUnits=deg  SpringStiffness=0  SpringStiffnessUnits=N*m/deg  DampingCoefficient=0  DampingCoefficientUnits=m^2*kg/s/rad  TorqueActuationMode=InputTorque  MotionActuationMode=ComputedMotion  SensePosition=on  SenseVelocity=on  SenseAcceleration=off  SenseTorqueForce=off  SenseLowerLimitTorqueForce=off  SenseUpperLimitTorqueForce=off  LowerLimitSpecify=on  LowerLimitBound=-3.14  LowerLimitBoundUnits=rad  LowerLimitStiffness=1e4  LowerLimitStiffnessUnits=N*m/deg  LowerLimitDamping=10  LowerLimitDampingUnits=N*m/(deg/s)  LowerLimitTransitionRegionWidth=0.1  LowerLimitTransitionRegionWidthUnits=deg  UpperLimitSpecify=on  UpperLimitBound=3.14  UpperLimitBoundUnits=rad  UpperLimitStiffness=1e4  UpperLimitStiffnessUnits=N*m/deg  UpperLimitDamping=10  UpperLimitDampingUnits=N*m/(deg/s)  UpperLimitTransitionRegionWidth=0.1  UpperLimitTransitionRegionWidthUnits=deg  PositionTargetSpecify=on  PositionTargetPriority=High  PositionTargetValue=0  PositionTargetValueUnits=rad  VelocityTargetSpecify=off  VelocityTargetPriority=High  VelocityTargetValue=0  VelocityTargetValueUnits=deg/s
  link1 : Subsystem
  link2 : Subsystem
  link3 : Subsystem
  link4 : Subsystem
  link5 : Subsystem
  link6 : Subsystem
  table : Subsystem
  tablefixed : sm_lib/Joints/Weld Joint  JointMode=Normal  SenseConstraintForce=off  SenseConstraintForceX=off  SenseConstraintForceY=off  SenseConstraintForceZ=off  SenseConstraintTorque=off  SenseConstraintTorqueX=off  SenseConstraintTorqueY=off  SenseConstraintTorqueZ=off  SenseTotalForce=off  SenseTotalForceX=off  SenseTotalForceY=off  SenseTotalForceZ=off  SenseTotalTorque=off  SenseTotalTorqueX=off  SenseTotalTorqueY=off  SenseTotalTorqueZ=off  CompositeWrenchDir=FollowerOnBase  CompositeWrenchFrame=BaseFrame
  input1 : PMIOPort  Side=Left
  input2 : PMIOPort  Port=2  Side=Left
  input3 : PMIOPort  Port=3  Side=Left
  input4 : PMIOPort  Port=4  Side=Left
  input5 : PMIOPort  Port=5  Side=Left
  input6 : PMIOPort  Port=6  Side=Left
  q : Outport
  dq : Outport  Port=2
  myT : Outport  Port=3
  v : Outport  Port=4
  wires:
  PS-Simulink Converter4/1 -> Mux/5
  PS-Simulink Converter2/1 -> Mux/3
  PS-Simulink Converter3/1 -> Mux/4
  PS-Simulink Converter5/1 -> Mux/6
  PS-Simulink Converter1/1 -> Mux/2
  PS-Simulink Converter8/1 -> Mux1/3
  PS-Simulink Converter9/1 -> Mux1/4
  PS-Simulink Converter6/1 -> Mux1/1
  PS-Simulink Converter10/1 -> Mux1/5
  PS-Simulink Converter7/1 -> Mux1/2
  PS-Simulink Converter11/1 -> Mux1/6
  PS-Simulink Converter/1 -> Mux/1
  Mux/1 -> q/1
  Mux1/1 -> dq/1
  PS-Simulink Converter27/1 -> Mux5/1
  PS-Simulink Converter29/1 -> Mux5/2
  PS-Simulink Converter26/1 -> Mux4/1
  MATLAB Function1/1(T) -> myT/1
  Mux5/1 -> v/1
  MATLAB Function/1(rpy) -> Display3/1
  Transpose/1 -> MATLAB Function1/1(R), MATLAB Function/1(Tr), Display2/1
  Mux4/1 -> Display1/1, MATLAB Function1/2(xyz)
  PS-Simulink Converter28/1 -> Transpose/1
  PS-Simulink Converter24/1 -> Mux4/3
  PS-Simulink Converter25/1 -> Mux4/2
  PS-Simulink Converter30/1 -> Mux5/3
  connections:
  joint2/LConn1 -- link1/RConn1
  end/LConn1 -- link6/RConn1
  joint1/RConn1 -- link1/LConn1
  joint5/LConn1 -- link4/RConn1
  PS-Simulink Converter5/LConn1 -- joint6/RConn2
  PS-Simulink Converter4/LConn1 -- joint5/RConn2
  joint5/RConn1 -- link5/LConn1
  joint2/RConn3 -- PS-Simulink Converter7/LConn1
  PS-Simulink Converter1/LConn1 -- joint2/RConn2
  joint2/RConn1 -- link2/LConn1
  end/RConn1 -- Transform Sensor1/LConn1 -- end1/LConn1
  joint6/RConn1 -- link6/LConn1
  PS-Simulink Converter3/LConn1 -- joint4/RConn2
  joint3/LConn1 -- link2/RConn1
  joint5/RConn3 -- PS-Simulink Converter10/LConn1
  joint3/RConn1 -- link3/LConn1
  joint6/RConn3 -- PS-Simulink Converter11/LConn1
  joint1/RConn3 -- PS-Simulink Converter6/LConn1
  joint4/RConn3 -- PS-Simulink Converter9/LConn1
  joint6/LConn1 -- link5/RConn1
  joint3/RConn3 -- PS-Simulink Converter8/LConn1
  MechanismConfiguration/RConn1 -- base_link/LConn1 -- World/RConn1 -- Solver Configuration/RConn1
  joint4/LConn1 -- link3/RConn1
  joint4/RConn1 -- link4/LConn1
  PS-Simulink Converter/LConn1 -- joint1/RConn2
  PS-Simulink Converter2/LConn1 -- joint3/RConn2
  joint4/LConn2 -- input4/RConn1
  joint3/LConn2 -- input3/RConn1
  joint1/LConn2 -- input1/RConn1
  joint2/LConn2 -- input2/RConn1
  joint5/LConn2 -- input5/RConn1
  joint6/LConn2 -- input6/RConn1
  PS-Simulink Converter24/LConn1 -- Transform Sensor1/RConn5
  PS-Simulink Converter26/LConn1 -- Transform Sensor1/RConn3
  PS-Simulink Converter29/LConn1 -- Transform Sensor1/RConn7
  PS-Simulink Converter25/LConn1 -- Transform Sensor1/RConn4
  Transform Sensor1/RConn6 -- PS-Simulink Converter27/LConn1
  Transform Sensor1/RConn2 -- PS-Simulink Converter28/LConn1
  Transform Sensor1/RConn8 -- PS-Simulink Converter30/LConn1
  base_link/RConn2 -- joint1/LConn1
  base_link/RConn1 -- tablefixed/LConn1
  table/LConn1 -- tablefixed/RConn1
